simulink model "FOCSpdTrq"  (R2023a)
settings: Solver=ode1  StartTime=0.0  StopTime=0.2  FixedStep=ctrlConst.TsSwitch  MaxStep=1e-6  RelTol=1e-3  EnableMultiTasking=on
undefined symbols (not defined in the file or in its folder): ECM, f32_P_SpdNeglimit_rpm, f32_P_SpdPoslimit_rpm, f32_P_SpeedPiMaxRatio, f32_P_SpeedPiMinRatio, g_msgCore0to2_alphaLow, g_msgCore0to2_Asrctrlmode, g_msgCore0to2_AsrKpHi, g_msgCore0to2_AsrKpLo, g_msgCore0to2_AsrKpZero, g_msgCore0to2_AsrSwtHiRpm, g_msgCore0to2_AsrSwtLoRpm, g_msgCore0to2_AsrTiHi, g_msgCore0to2_AsrTiLo, g_msgCore0to2_AsrTiZero, g_msgCore0to2_betaLow, g_msgCore0to2_CalibEn2, g_msgCore0to2_coeff, g_msgCore0to2_cos_Amp, g_msgCore0to2_cos_frq, g_msgCore0to2_cos_phase, g_msgCore0to2_frqfix_K, g_msgCore0to2_H_coef, g_msgCore0to2_HFcoef, g_msgCore0to2_K1, g_msgCore0to2_K1switch, g_msgCore0to2_K2, g_msgCore0to2_K3, g_msgCore0to2_K3switch, g_msgCore0to2_Kvp, g_msgCore0to2_L_coef, g_msgCore0to2_LFcoef, g_msgCore0to2_LPF_coef, g_msgCore0to2_maxCur2, g_msgCore0to2_maxTrq2, g_msgCore0to2_R_Kr, g_msgCore0to2_R_outputGain, g_msgCore0to2_R_Outputlimit, g_msgCore0to2_R_Wc, g_msgCore0to2_Rswitch, g_msgCore0to2_sin_Amp, g_msgCore0to2_sin_frq, g_msgCore0to2_sin_phase, g_msgCore0to2_Trqfix, g_msgCoreoto2_R_woGain
libraries: simulink x2
settings Model: Creator=M00039784  LastModifiedBy=HP
settings SolverCC: AlgebraicLoopSolver=TrustRegion  InsertRTBMode=Never (minimum delay)
settings DataIOCC: LimitDataPoints=on  SaveFormat=Array  SaveOutput=off  SaveTime=off
settings OptimizationCC: DefaultParameterBehavior=Inlined  UseDivisionForNetSlopeComputation=on  UseFloatMulNetSlope=on  DefaultUnderspecifiedDataType=single  InlineInvariantSignals=on  ReuseModelBlockBuffer=off  PassReuseOutputArgsAs=Individual arguments  ExpressionDepthLimit=2147483647  ZeroExternalMemoryAtStartup=off  ZeroInternalMemoryAtStartup=off  NoFixptDivByZeroProtection=on  EfficientFloat2IntCast=on  LifeSpan=1  EfficientTunableParamExpr=on
settings DebuggingCC: ReadBeforeWriteMsg=DisableAll  WriteAfterWriteMsg=DisableAll  WriteAfterReadMsg=DisableAll  AlgebraicLoopMsg=none  MultiTaskDSMMsg=none  SingleTaskRateTransMsg=error  IntegerOverflowMsg=none  ParameterPrecisionLossMsg=none  BusObjectLabelMismatch=none  AssertControl=DisableAll  AllowSymbolicDim=off  StateNameClashWarn=warning  SFUnexpectedBacktrackingDiag=warning  SFNoUnconditionalDefaultTransitionDiag=warning  SFExecutionAtInitializationDiag=none  IntegerSaturationMsg=none  UnitsInconsistencyMsg=none  ArithmeticOperatorsInVariantConditions=warning
settings HardwareCC: ProdBitPerPointer=32  ProdBitPerSizeT=32  ProdBitPerPtrDiffT=32  ProdLargestAtomicFloat=None  ProdWordSize=32  ProdHWDeviceType=Infineon->TriCore
settings ModelReferenceCC: UpdateModelReferenceTargets=IfOutOfDate  EnableRefExpFcnMdlSchedulingChecks=on  ModelReferenceNumInstancesAllowed=Single  PropagateSignalLabelsOutOfModel=off
settings SFSimCC: SFSimEcho=off  SimUseLocalCustomCode=off  SimGenImportedTypeDefs=on  MATLABDynamicMemAlloc=off  CustomCodeUndefinedFunction=UseInterfaceOnly
settings RTWCC: Description=Embedded Coder  SystemTargetFile=ert.tlc  GenCodeOnly=on  GenerateMakefile=off  TemplateMakefile=ec_target.tmf  RTWVerbose=off  RTWUseLocalCustomCode=off  CodeExecutionProfiling=on  CodeProfilingSaveOptions=AllData  CodeProfilingInstrumentation=detailed
settings CodeAppCC: ForceParamTrailComments=on  IgnoreCustomStorageClasses=off  IgnoreTestpoints=on  MaxIdLength=64  SimulinkDataObjDesc=on  MATLABFcnDesc=on  CustomSymbolStrGlobalVar=GRS$N$M  CustomSymbolStrType=pmsmfocS_$N$M  CustomSymbolStrFcn=$N$M$F  CustomSymbolStrFcnArg=$I$N$M  CustomSymbolStrMacro=$N$M  InsertBlockDesc=on  StateflowObjectComments=on  MATLABSourceComments=on  InternalIdentifier=Classic
settings ERTTargetCC: TargetLangStandard=C99 (ISO)  UtilityFuncGeneration=Shared location  MultiwordLength=2048  CombineSignalStateStructs=on  SupportAbsoluteTime=off  SupportNonFinite=off  SupportComplex=off  SupportNonInlinedSFcns=on  RemoveResetFunc=off  ParenthesesLevel=Maximum  GenerateASAP2=on  InlinedParameterPlacement=NonHierarchical  ERTCustomFileTemplate=example_file_process.tlc  EnableDataOwnership=on  ConvertIfToSwitch=off  SuppressUnreachableDefaultCases=off  MemSecPackage=Simulink  MemSecDataConstants=MemConst  MemSecDataParameters=MemConstVolatile
settings ConfigComp: CovMetricSettings=dcmtrzow  CovHTMLOptions=-aTS=1 -bRG=1 -bTC=1 -hTR=0 -nFC=0 -scm=1 -bcm=1 -xEv=0  CovSaveCumulativeToWorkspaceVar=on  CovSaveSingleToWorkspaceVar=on  CovExternalEMLEnable=off  CovSFcnEnable=off
settings SimscapeCC: SimscapeNormalizeSystem=off

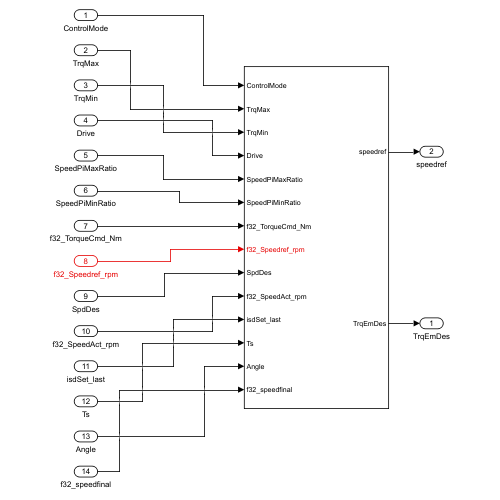
[thumbnail: Simulink's stored preview of the top-level diagram]
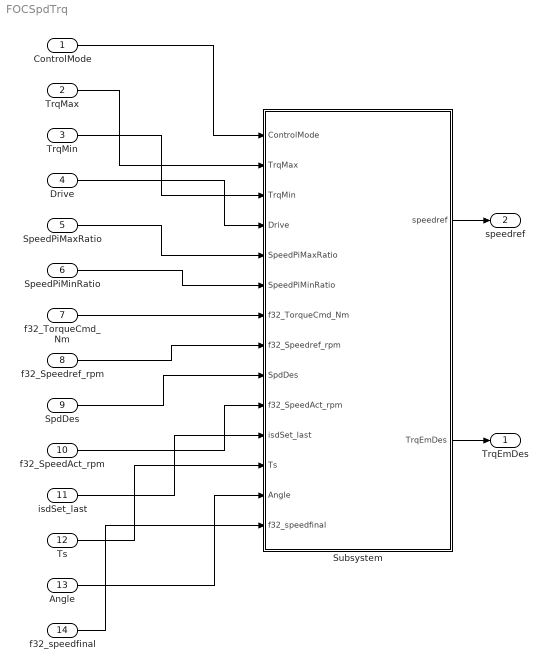
== system FOCSpdTrq ==
  ControlMode : Inport  OutDataTypeStr=Enum: ECM  PortDimensions=1  SampleTime=0.0001
  TrqMax : Inport  Port=2
  TrqMin : Inport  Port=3
  Drive : Inport  Port=4
  SpeedPiMaxRatio : Inport  Port=5
  SpeedPiMinRatio : Inport  Port=6
  f32_TorqueCmd_Nm : Inport  Port=7  OutDataTypeStr=single  PortDimensions=1
  f32_Speedref_rpm : Inport  Port=8  OutDataTypeStr=single  PortDimensions=1  SampleTime=0.0001
  SpdDes : Inport  Port=9
  f32_SpeedAct_rpm : Inport  Port=10  OutDataTypeStr=single  PortDimensions=1  SampleTime=0.0001
  isdSet_last : Inport  Port=11
  Ts : Inport  Port=12
  Angle : Inport  Port=13  OutDataTypeStr=int16  PortDimensions=1  SampleTime=0.0001
  f32_speedfinal : Inport  Port=14
  Subsystem : Subsystem
  TrqEmDes : Outport
  speedref : Outport  Port=2
  wires:
  SpeedPiMaxRatio/1 -> Subsystem/5(SpeedPiMaxRatio)
  SpdDes/1 -> Subsystem/9(SpdDes)
  ControlMode/1 -> Subsystem/1(ControlMode)
  SpeedPiMinRatio/1 -> Subsystem/6(SpeedPiMinRatio)
  TrqMax/1 -> Subsystem/2(TrqMax)
  f32_TorqueCmd_Nm/1 -> Subsystem/7(f32_TorqueCmd_Nm)
  TrqMin/1 -> Subsystem/3(TrqMin)
  f32_Speedref_rpm/1 -> Subsystem/8(f32_Speedref_rpm)
  Drive/1 -> Subsystem/4(Drive)
  f32_SpeedAct_rpm/1 -> Subsystem/10(f32_SpeedAct_rpm)
  isdSet_last/1 -> Subsystem/11(isdSet_last)
  Ts/1 -> Subsystem/12(Ts)
  Angle/1 -> Subsystem/13(Angle)
  f32_speedfinal/1 -> Subsystem/14(f32_speedfinal)
  Subsystem/1(speedref) -> speedref/1
  Subsystem/2(TrqEmDes) -> TrqEmDes/1

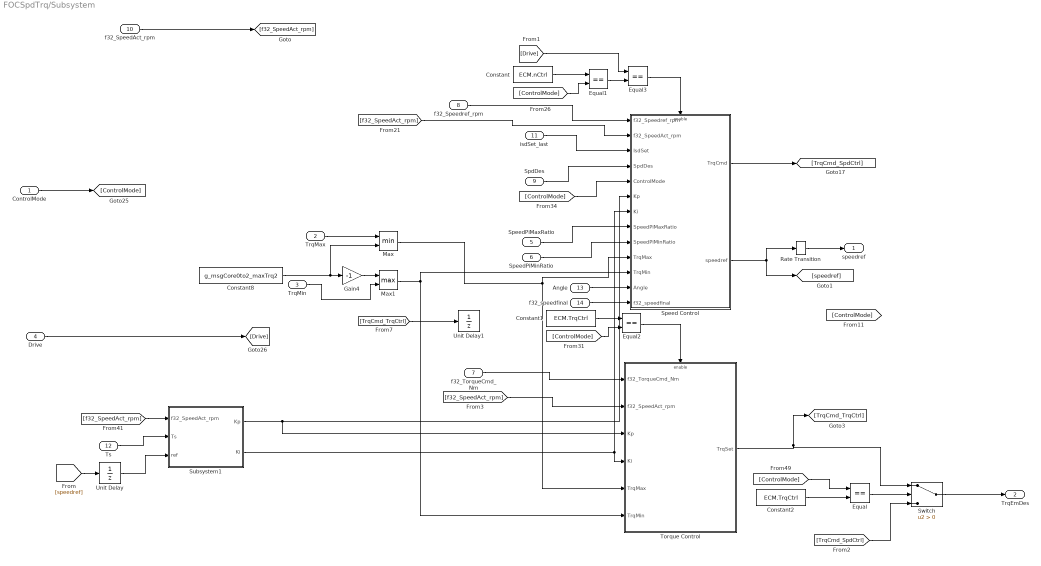
== system FOCSpdTrq/Subsystem ==
  ControlMode : Inport  OutDataTypeStr=Enum: ECM  PortDimensions=1  SampleTime=0.0001
  TrqMax : Inport  Port=2
  TrqMin : Inport  Port=3
  Drive : Inport  Port=4
  SpeedPiMaxRatio : Inport  Port=5
  SpeedPiMinRatio : Inport  Port=6
  f32_TorqueCmd_Nm : Inport  Port=7  OutDataTypeStr=single  PortDimensions=1
  f32_Speedref_rpm : Inport  Port=8  OutDataTypeStr=single  PortDimensions=1  SampleTime=0.0001
  SpdDes : Inport  Port=9
  f32_SpeedAct_rpm : Inport  Port=10  OutDataTypeStr=single  PortDimensions=1  SampleTime=0.0001
  isdSet_last : Inport  Port=11
  Ts : Inport  Port=12
  Angle : Inport  Port=13  OutDataTypeStr=int16  PortDimensions=1  SampleTime=0.0001
  f32_speedfinal : Inport  Port=14
  Constant : Constant  Value=ECM.nCtrl
  Constant1 : Constant  Value=ECM.TrqCtrl
  Constant2 : Constant  Value=ECM.TrqCtrl
  Constant8 : Constant  Value=g_msgCore0to2_maxTrq2  OutDataTypeStr=single  SampleTime=-1
  Equal{,1..3} (4 alike) : RelationalOperator  Operator===  OutDataTypeStr=boolean  RndMeth=Simplest  InputSameDT=off
  Gain4 : Gain  Gain=-1
  Max : MinMax  Inputs=2
  Max1 : MinMax  Function=max  Inputs=2
  Rate Transition : RateTransition
  Speed Control : Subsystem
  Subsystem1 : Subsystem
  Switch : Switch  Criteria=u2 > Threshold  SaturateOnIntegerOverflow=off  InputSameDT=off
  Torque Control : Subsystem
  Unit Delay : UnitDelay  SampleTime=-1  HasFrameUpgradeWarning=on
  Unit Delay1 : UnitDelay  SampleTime=-1  HasFrameUpgradeWarning=on
  speedref : Outport
  TrqEmDes : Outport  Port=2
  wires:
  isdSet_last/1 -> Speed Control/3(IsdSet)
  f32_Speedref_rpm/1 -> Speed Control/1(f32_Speedref_rpm)
  [ControlMode] -> Speed Control/5(ControlMode)
  Subsystem1/1(Kp) -> Speed Control/6(Kp), Torque Control/3(Kp)
  Equal1/1 -> Equal3/2
  Speed Control/1("TrqCmd ") -> [TrqCmd_SpdCtrl]
  Constant2/1 -> Equal/2
  SpeedPiMinRatio/1 -> Speed Control/9(SpeedPiMinRatio)
  [ControlMode] -> Equal/1
  Torque Control/1(TrqSet) -> Switch/1, [TrqCmd_TrqCtrl]
  Max/1 -> Speed Control/10(TrqMax), Torque Control/5(TrqMax)
  [Drive] -> Equal3/1
  Max1/1 -> Torque Control/6(TrqMin), Speed Control/11(TrqMin)
  [f32_SpeedAct_rpm] -> Speed Control/2(f32_SpeedAct_rpm)
  [f32_SpeedAct_rpm] -> Torque Control/2(f32_SpeedAct_rpm)
  SpeedPiMaxRatio/1 -> Speed Control/8(SpeedPiMaxRatio)
  Equal/1 -> Switch/2
  [ControlMode] -> Equal2/2
  Switch/1 -> TrqEmDes/1
  [ControlMode] -> Equal1/2
  TrqMin/1 -> Max1/2
  Subsystem1/2(Ki) -> Speed Control/7(Ki), Torque Control/4(Ki)
  ControlMode/1 -> [ControlMode]
  [TrqCmd_SpdCtrl] -> Switch/3
  Constant1/1 -> Equal2/1
  Drive/1 -> [Drive]
  [f32_SpeedAct_rpm] -> Subsystem1/1(f32_SpeedAct_rpm)
  Ts/1 -> Subsystem1/2(Ts)
  Constant/1 -> Equal1/1
  SpdDes/1 -> Speed Control/4(SpdDes)
  Equal2/1 -> Torque Control/Enable
  Gain4/1 -> Max1/1
  Constant8/1 -> Max/2, Gain4/1
  TrqMax/1 -> Max/1
  f32_SpeedAct_rpm/1 -> [f32_SpeedAct_rpm]
  Equal3/1 -> Speed Control/Enable
  Speed Control/2(speedref) -> Rate Transition/1, [speedref]
  f32_TorqueCmd_Nm/1 -> Torque Control/1(f32_TorqueCmd_Nm)
  [TrqCmd_TrqCtrl] -> Unit Delay1/1
  Angle/1 -> Speed Control/12(Angle)
  [speedref] -> Unit Delay/1
  Unit Delay/1 -> Subsystem1/3(ref)
  f32_speedfinal/1 -> Speed Control/13(f32_speedfinal)
  Rate Transition/1 -> speedref/1

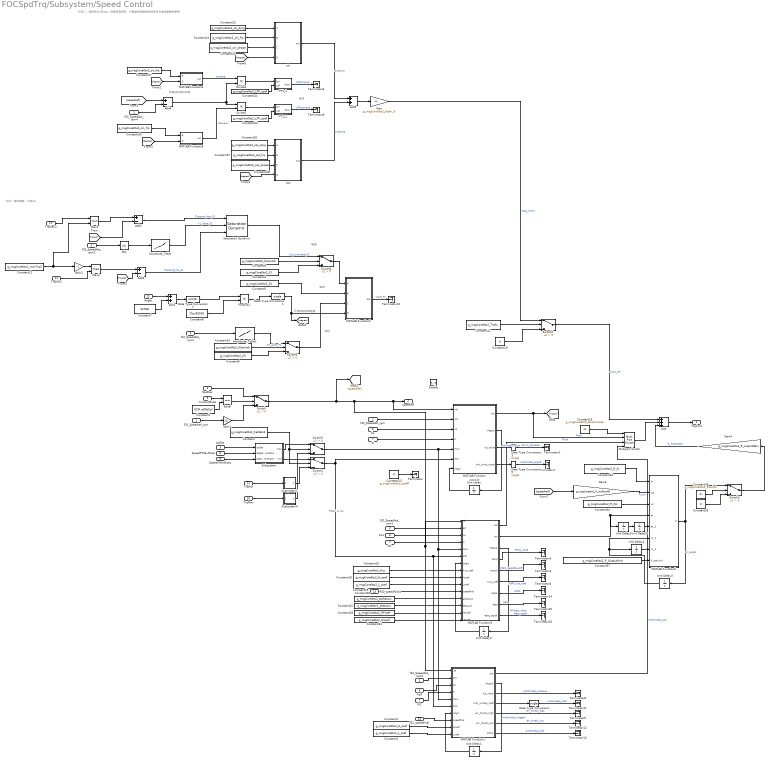
== system FOCSpdTrq/Subsystem/Speed Control ==
  note: PDFF & Up
  note: 幅值
  note: 方法二，同时有sin和cos，但是没有闭环，只把坐标变换后的信号作为调试参数的参考
  note: 方法一波动抑制，只有sin
  note: 去除系数
  note: 频率·
  note: 相位
  note: 外部接收机械角度
  note: 转速波动坐标变换
  note: 滤波
  f32_Speedref_rpm : Inport
  f32_SpeedAct_rpm : Inport  Port=2
  IsdSet : Inport  Port=3
  SpdDes : Inport  Port=4
  ControlMode : Inport  Port=5
  Kp : Inport  Port=6
  Ki : Inport  Port=7
  SpeedPiMaxRatio : Inport  Port=8
  SpeedPiMinRatio : Inport  Port=9
  TrqMax : Inport  Port=10
  TrqMin : Inport  Port=11
  Angle : Inport  Port=12  OutDataTypeStr=int16  PortDimensions=1  SampleTime=0.0001
  f32_speedfinal : Inport  Port=13
  Enable : EnablePort  StatesWhenEnabling=reset
  Abs : Abs  SaturateOnIntegerOverflow=off
  Add : Sum  Inputs=+++
  Add1 : Sum  OutDataTypeStr=int16
  Add2 : Sum  Inputs=+-
  Add3 : Sum  Inputs=+-
  Add4 : Sum  Inputs=+-
  Add5 : Sum
  Amplitude_Table : Lookup_n-D  NumberOfTableDimensions=1  DataSpecification=Lookup table object  LookupTableObject=cripple_T_P1  BreakpointsForDimension1=|  BeginIndexSearchUsingPreviousIndexResult=on  Table=|  ExtrapMethod=Clip  UseLastTableValue=on  InternalRulePriority=Speed  OutDataTypeStr=Inherit: Inherit from 'Table data'
      BreakpointsForDimension1=|
      | [-530.4101839
      | -495.049505
      | -459.688826
      | -424.3281471
      | -388.9674682
      | -353.6067893
      | -318.2461103
      | -282.8854314
      | -247.5247525
      | -212.1640736
      | -176.8033946
      | -141.4427157
      | -106.0820368
      | -70.72135785
      | -35.36067893
      | 0
      | 35.36067893
      | 70.72135785
      | 106.0820368
      | 141.4427157
      | 176.8033946
      | 212.1640736
      | 247.5247525
      | 282.8854314
      | 318.2461103
      | 353.6067893
      | 388.9674682
      | 424.3281471
      | 459.688826
      | 495.049505
      | 530.4101839
      | ]
      Table=|
      | [0.983333333
      | 0.983333333
      | 0.985185185
      | 0.987037037
      | 0.990740741
      | 0.992592593
      | 0.994444444
      | 0.996296296
      | 0.996296296
      | 0.998148148
      | 0.998148148
      | 0.998148148
      | 0.994444444
      | 0.992592593
      | 0.990740741
      | 0.990740741
      | 0.990740741
      | 0.992592593
      | 0.996296296
      | 1
      | 1
      | 1
      | 1
      | 0.998148148
      | 0.996296296
      | 0.994444444
      | 0.992592593
      | 0.990740741
      | 0.988888889
      | 0.987037037
      | 0.987037037]
  Amplitude_Table1 : Lookup_n-D  NumberOfTableDimensions=1  DataSpecification=Lookup table object  LookupTableObject=cphase_T_P1  BreakpointsForDimension1=|  BeginIndexSearchUsingPreviousIndexResult=on  Table=|  ExtrapMethod=Clip  UseLastTableValue=on  InternalRulePriority=Speed  OutDataTypeStr=Inherit: Inherit from 'Table data'
      BreakpointsForDimension1=|
      | [-530.4101839
      | -495.049505
      | -459.688826
      | -424.3281471
      | -388.9674682
      | -353.6067893
      | -318.2461103
      | -282.8854314
      | -247.5247525
      | -212.1640736
      | -176.8033946
      | -141.4427157
      | -106.0820368
      | -70.72135785
      | -35.36067893
      | 0
      | 35.36067893
      | 70.72135785
      | 106.0820368
      | 141.4427157
      | 176.8033946
      | 212.1640736
      | 247.5247525
      | 282.8854314
      | 318.2461103
      | 353.6067893
      | 388.9674682
      | 424.3281471
      | 459.688826
      | 495.049505
      | 530.4101839
      | ]
      Table=|
      | [0.983333333
      | 0.983333333
      | 0.985185185
      | 0.987037037
      | 0.990740741
      | 0.992592593
      | 0.994444444
      | 0.996296296
      | 0.996296296
      | 0.998148148
      | 0.998148148
      | 0.998148148
      | 0.994444444
      | 0.992592593
      | 0.990740741
      | 0.990740741
      | 0.990740741
      | 0.992592593
      | 0.996296296
      | 1
      | 1
      | 1
      | 1
      | 0.998148148
      | 0.996296296
      | 0.994444444
      | 0.992592593
      | 0.990740741
      | 0.988888889
      | 0.987037037
      | 0.987037037]
  Constant : Constant  Value=g_msgCore0to2_CalibEn2
  Constant1 : Constant  Value=g_msgCore0to2_H_coef
  Constant10 : Constant  Value=0  OutDataTypeStr=single
  Constant11 : Constant  Value=g_msgCore0to2_Trqfix  OutDataTypeStr=single
  Constant12 : Constant  Value=g_msgCore0to2_maxTrq2  OutDataTypeStr=single  SampleTime=-1
  Constant13 : Constant  Value=g_msgCore0to2_coeff  OutDataTypeStr=single
  Constant14 : Constant  Value=g_msgCore0to2_K3switch
  Constant15 : Constant  Value=g_msgCore0to2_Kvp
  Constant16 : Constant  Value=g_msgCore0to2_Asrctrlmode
  Constant17 : Constant  Value=g_msgCore0to2_sin_frq
  Constant18 : Constant  Value=g_msgCore0to2_H_coef
  Constant19 : Constant  Value=g_msgCore0to2_L_coef
  Constant2 : Constant  Value=ECM.alOfsCal
  Constant20 : Constant  Value=g_msgCore0to2_alphaLow
  Constant21 : Constant  Value=g_msgCore0to2_LPF_coef  OutDataTypeStr=single
  Constant22 : Constant  Value=g_msgCore0to2_LPF_coef  OutDataTypeStr=single
  Constant23 : Constant  Value=g_msgCore0to2_sin_Amp
  Constant24 : Constant  Value=g_msgCore0to2_sin_frq
  Constant25 : Constant  Value=g_msgCore0to2_sin_phase
  Constant26 : Constant  Value=g_msgCore0to2_cos_Amp
  Constant27 : Constant  Value=g_msgCore0to2_cos_frq
  Constant28 : Constant  Value=g_msgCore0to2_cos_phase
  Constant29 : Constant  Value=g_msgCore0to2_HFcoef
  Constant3 : Constant  Value=g_msgCore0to2_L_coef
  Constant30 : Constant  Value=g_msgCore0to2_sin_frq
  Constant31 : Constant  Value=g_msgCore0to2_LFcoef
  Constant32 : Constant  Value=g_msgCore0to2_betaLow
  Constant33 : Constant  Value=g_msgCore0to2_R_Kr
  Constant34 : Constant  Value=g_msgCore0to2_R_Wc
  Constant35 : Constant  Value=0
  Constant36 : Constant  Value=g_msgCore0to2_Rswitch
  Constant37 : Constant  Value=g_msgCore0to2_R_Outputlimit
  Constant4 : Constant  Value=g_msgCore0to2_K1
  Constant5 : Constant  Value=g_msgCore0to2_K2
  Constant6 : Constant  Value=g_msgCore0to2_K3
  Constant7 : Constant  Value=32768  OutDataTypeStr=int16
  Constant8 : Constant  Value=2*pi/65535  OutDataTypeStr=single
  Constant9 : Constant  Value=g_msgCore0to2_K1switch
  Data Type Conversion{,1,3,5} (4 alike) : DataTypeConversion  OutDataTypeStr=single  SaturateOnIntegerOverflow=off  RndMeth=Floor
  Data Type Conversion2 : DataTypeConversion  OutDataTypeStr=uint16  SaturateOnIntegerOverflow=off  RndMeth=Floor
  Divide1 : Product  Inputs=**  OutDataTypeStr=single
  Divide2 : Product  Inputs=**  OutDataTypeStr=single
  Equal : RelationalOperator  Operator===  OutDataTypeStr=boolean  RndMeth=Simplest  InputSameDT=off
  Gain : Gain  Gain=g_msgCore0to2_frqfix_K
  Gain1 : Gain  Gain=12
  Gain2 : Gain  Gain=-1
  Gain3 : Gain  Gain=g_msgCoreoto2_R_woGain/60
  Gain4 : Gain  Gain=g_msgCore0to2_R_outputGain  OutDataTypeStr=single
  Ki1 : InportShadow  Port=7
  Ki2 : InportShadow  Port=7
  Kp1 : InportShadow  Port=6
  Kp3 : InportShadow  Port=6
  MATLAB Function : MATLAB Function  TreatAsAtomicUnit=on
  MATLAB Function1 : MATLAB Function  TreatAsAtomicUnit=on
  MATLAB Function2 : MATLAB Function  TreatAsAtomicUnit=on
  MATLAB Function3 : MATLAB Function  TreatAsAtomicUnit=on
  MATLAB Function4 : MATLAB Function  TreatAsAtomicUnit=on
  MATLAB Function5 : MATLAB Function  TreatAsAtomicUnit=on
  MATLAB Function6 : MATLAB Function  TreatAsAtomicUnit=on
  Max2 : MinMax  Inputs=2
  Max3 : MinMax  Function=max  Inputs=2
  Multiport Switch : MultiPortSwitch  SaturateOnIntegerOverflow=off  InputSameDT=off
  PT1_1 : Subsystem
  PT1_2 : Subsystem
  Product1 : Product  OutDataTypeStr=single
  Saturation Dynamic : simulink/Discontinuities/Saturation Dynamic  OutMin=[]  OutMax=[]  OutDataTypeStr=Inherit: Same as second input  OutDataType=fixdt(1, 16)  OutScaling=2^-10  DoSatur=off
  Subsystem : Subsystem
  Subsystem1 : Subsystem
  Subsystem4 : Subsystem
  Switch{,1..6} (7 alike) : Switch  Criteria=u2 > Threshold  SaturateOnIntegerOverflow=off  InputSameDT=off
  Terminator{,1..16} (17 alike) : Terminator
  TrqMax2 : InportShadow  Port=10
  TrqMin2 : InportShadow  Port=11
  Unit Delay{,1..6} (7 alike) : UnitDelay  SampleTime=-1  HasFrameUpgradeWarning=on
  cos : MATLAB Function  TreatAsAtomicUnit=on
  f32_SpeedAct_rpm{1..5} (5 alike) : InportShadow  Port=2
  f32_speedfinal1 : InportShadow  Port=13
  "sin " : MATLAB Function  TreatAsAtomicUnit=on
  "TrqCmd " : Outport  OutputWhenDisabled=reset  InitialOutput=0
  speedref : Outport  Port=2  OutputWhenDisabled=reset  InitialOutput=0
  wires:
  IsdSet/1 -> Subsystem/1(IsdSet)
  Switch2/1 -> MATLAB Function/6(MIN), MATLAB Function1/6(MIN), MATLAB Function3/6(MIN)
  Switch1/1 -> MATLAB Function/5(MAX), MATLAB Function1/5(MAX), MATLAB Function3/5(MAX)
  f32_SpeedAct_rpm/1 -> MATLAB Function/2(act)
  Switch/1 -> [speedref], MATLAB Function1/1(ref), MATLAB Function3/1(ref), MATLAB Function/1(ref), speedref/1
  MATLAB Function/2(intgout) -> Unit Delay/1  "Asrintgin_value"
  ControlMode/1 -> Equal/1
  Equal/1 -> Switch/2
  SpdDes/1 -> Switch/1
  f32_Speedref_rpm/1 -> Gain1/1
  Constant2/1 -> Equal/2
  Gain1/1 -> Switch/3
  Kp/1 -> MATLAB Function/3(kp)
  Ki/1 -> MATLAB Function/4(ki)
  SpeedPiMaxRatio/1 -> Subsystem/2(SpeedPiMaxRatio)
  SpeedPiMinRatio/1 -> Subsystem/3(SpeedPiMinRatio)
  Subsystem/1(max) -> Switch1/1
  Subsystem/2(min) -> Switch2/1
  Constant/1 -> Switch1/2, Switch2/2
  TrqMin/1 -> Subsystem1/1(" ")
  TrqMax/1 -> Subsystem4/1(" ")
  Subsystem4/1(Outport) -> Switch1/3
  Subsystem1/1(Outport) -> Switch2/3
  Unit Delay/1 -> MATLAB Function/7(intgin)
  Switch6/1 -> MATLAB Function2/3(C)
  Max3/1 -> Add3/1
  Constant12/1 -> Gain2/1, Max2/2
  Saturation Dynamic/1 -> Switch4/1  "K1_Limitvalue_P1"
  f32_SpeedAct_rpm3/1 -> Abs/1
  [Trqspd] -> Add2/2
  Amplitude_Table/1 -> Saturation Dynamic/2  "K1_value_P1"
  Add3/1 -> Saturation Dynamic/3  "Trqcomp_Min_P1"
  [Trqspd] -> Add3/2
  Switch5/1 -> Add/1  "comp_P1"
  Max2/1 -> Add2/1
  Constant9/1 -> Switch4/2
  Constant14/1 -> Switch6/2
  Constant8/1 -> Product1/2
  Constant7/1 -> Add1/2
  Constant6/1 -> Switch6/3
  TrqMin2/1 -> Max3/2
  Constant4/1 -> Switch4/3
  Gain2/1 -> Max3/1
  Constant10/1 -> Switch5/3
  Constant5/1 -> MATLAB Function2/2(B)
  Add2/1 -> Saturation Dynamic/1  "Trqcomp_Max_P1"
  Angle/1 -> Add1/1
  Abs/1 -> Amplitude_Table/1
  Constant11/1 -> Switch5/2
  Data Type Conversion1/1 -> [degree], MATLAB Function2/4(D)
  f32_SpeedAct_rpm2/1 -> Amplitude_Table1/1
  Product1/1 -> Data Type Conversion1/1
  Amplitude_Table1/1 -> Switch6/1  "K3_value_P1"
  Switch4/1 -> MATLAB Function2/1(A)
  Add1/1 -> Data Type Conversion2/1
  Data Type Conversion2/1 -> Product1/1
  Add/1 -> "TrqCmd "/1
  TrqMax2/1 -> Max2/1
  MATLAB Function/1(out) -> Multiport Switch/2, [Trqspd]  "PIout"
  MATLAB Function/3(Kp_value) -> Data Type Conversion3/1
  Constant16/1 -> Multiport Switch/1
  MATLAB Function3/1(out) -> Multiport Switch/3  "FFout"
  MATLAB Function3/3(intgout) -> Unit Delay2/1  "FFintgin_value"
  Unit Delay2/1 -> MATLAB Function3/7(intgin)
  f32_SpeedAct_rpm1/1 -> MATLAB Function3/2(act)
  Ki1/1 -> MATLAB Function3/4(ki)
  Kp1/1 -> MATLAB Function3/3(kp)
  Data Type Conversion3/1 -> Terminator1/1  "AsrKp_Calvalue"
  MATLAB Function3/4(temp) -> Terminator3/1  "FFKp_value"
  [speedref] -> Add4/1
  f32_SpeedAct_rpm4/1 -> Add4/2
  [degree] -> MATLAB Function4/2(D)
  [degree] -> MATLAB Function5/2(D)
  MATLAB Function4/1(out) -> Divide1/1  "sinwave"
  Add4/1 -> Divide2/1, Divide1/2
  MATLAB Function5/1(out) -> Divide2/2  "coswave"
  Divide1/1 -> PT1_1/1(bin)
  Constant21/1 -> PT1_1/2(cof)
  Divide2/1 -> PT1_2/1(bin)
  Constant22/1 -> PT1_2/2(cof)
  "sin "/1(out) -> Add5/1  "sinfixtrq"
  cos/1(out) -> Add5/2  "cosfixtrq"
  Add5/1 -> Gain/1
  [degree] -> cos/4(D)
  [degree] -> "sin "/4(D)
  Constant23/1 -> "sin "/1(A)
  Constant24/1 -> "sin "/2(B)
  Constant25/1 -> "sin "/3(C)
  Constant26/1 -> cos/1(A)
  Constant27/1 -> cos/2(B)
  Constant28/1 -> cos/3(C)
  Constant17/1 -> MATLAB Function4/1(B)
  Constant30/1 -> MATLAB Function5/1(B)
  Gain/1 -> Switch5/1  "total_fixtrq"
  Constant13/1 -> Terminator/1
  PT1_1/1(bout) -> Terminator6/1  "LPFsinwave"
  PT1_2/1(bout) -> Terminator9/1  "LPFcoswave"
  MATLAB Function2/1(out) -> Terminator10/1  "wave_P1"
  Kp3/1 -> MATLAB Function1/3(kp)
  Ki2/1 -> MATLAB Function1/4(ki)
  f32_SpeedAct_rpm5/1 -> MATLAB Function1/2(act)
  Unit Delay1/1 -> MATLAB Function1/7(intgin)
  MATLAB Function1/2(intgout) -> Unit Delay1/1  "AntiWindup_integral"
  MATLAB Function1/3(Kp_value) -> Terminator8/1  "AntiWindup_Kpvalue"
  MATLAB Function1/4(Anti_windup_coef) -> Data Type Conversion/1
  Data Type Conversion/1 -> Terminator11/1  "AntiWindup_coef"
  Multiport Switch/1 -> Add/2
  MATLAB Function1/1(out) -> Multiport Switch/4  "AntiWindup_out"
  MATLAB Function/4(Anti_wind_signal) -> Data Type Conversion5/1
  Data Type Conversion5/1 -> Terminator7/1  "AntiWindup_Signal"
  f32_speedfinal/1 -> MATLAB Function1/8(speedfinal)
  Constant1/1 -> MATLAB Function1/9(Hcoef)
  Constant3/1 -> MATLAB Function1/10(Lcoef)
  MATLAB Function1/5(err_thresh_high) -> Terminator5/1  "err_thresh_high"
  MATLAB Function1/6(err_thresh_low) -> Terminator12/1  "err_thresh_low"
  MATLAB Function1/7(alpha) -> Terminator13/1  "AntiWindup_Alfa"
  MATLAB Function3/5(temp1) -> Terminator2/1  "PDFF_SpdrefMuxKff"
  MATLAB Function3/6(Kvp_coef) -> Terminator4/1  "PDFF_Kvp_coef"
  Constant15/1 -> MATLAB Function3/8("Kvp_coef ")
  Constant18/1 -> MATLAB Function3/9(Hcoef)
  Constant19/1 -> MATLAB Function3/10(Lcoef)
  f32_speedfinal1/1 -> MATLAB Function3/11(speedfinal)
  Constant20/1 -> MATLAB Function3/12(alphaLow)
  MATLAB Function3/7(alpha) -> Terminator14/1  "alpha"
  Constant32/1 -> MATLAB Function3/13(betaLow)
  Constant29/1 -> MATLAB Function3/14(HFcoef)
  Constant31/1 -> MATLAB Function3/15(LFcoef)
  MATLAB Function3/8(beta) -> Terminator15/1  "beta"
  MATLAB Function3/9(beta_signal) -> Terminator16/1  "beta_signal"
  MATLAB Function6/1(yk) -> Unit Delay3/1, Switch3/1  "R_output"
  Unit Delay4/1 -> MATLAB Function6/7(yk_2)
  Unit Delay3/1 -> Unit Delay4/1, MATLAB Function6/6(yk_1)
  MATLAB Function3/2(err) -> Unit Delay6/1, MATLAB Function6/4(ek)
  Unit Delay5/1 -> MATLAB Function6/5(ek_2)
  Unit Delay6/1 -> Unit Delay5/1
  [speedref] -> Gain3/1
  Gain3/1 -> MATLAB Function6/2(w0)  "R_wo"
  Constant33/1 -> MATLAB Function6/1(Kr)
  Constant34/1 -> MATLAB Function6/3(wc)
  Switch3/1 -> Gain4/1
  Constant35/1 -> Switch3/3
  Constant36/1 -> Switch3/2
  Gain4/1 -> Add/3  "R_finaloutput"
  Constant37/1 -> MATLAB Function6/8(R_optLimt)

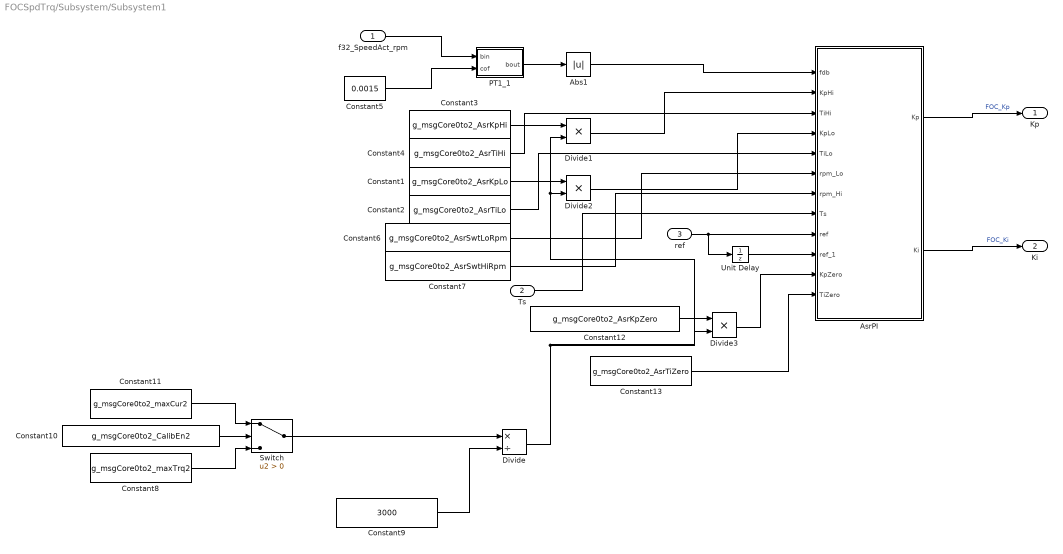
== system FOCSpdTrq/Subsystem/Subsystem1 ==
  f32_SpeedAct_rpm : Inport
  Ts : Inport  Port=2
  ref : Inport  Port=3
  Abs1 : Abs  SaturateOnIntegerOverflow=off
  AsrPI : MATLAB Function
  Constant1 : Constant  Value=g_msgCore0to2_AsrKpLo
  Constant10 : Constant  Value=g_msgCore0to2_CalibEn2
  Constant11 : Constant  Value=g_msgCore0to2_maxCur2  OutDataTypeStr=single  SampleTime=-1
  Constant12 : Constant  Value=g_msgCore0to2_AsrKpZero
  Constant13 : Constant  Value=g_msgCore0to2_AsrTiZero
  Constant2 : Constant  Value=g_msgCore0to2_AsrTiLo
  Constant3 : Constant  Value=g_msgCore0to2_AsrKpHi
  Constant4 : Constant  Value=g_msgCore0to2_AsrTiHi
  Constant5 : Constant  Value=0.0015  OutDataTypeStr=single
  Constant6 : Constant  Value=g_msgCore0to2_AsrSwtLoRpm
  Constant7 : Constant  Value=g_msgCore0to2_AsrSwtHiRpm
  Constant8 : Constant  Value=g_msgCore0to2_maxTrq2  OutDataTypeStr=single  SampleTime=-1
  Constant9 : Constant  Value=3000  OutDataTypeStr=single  SampleTime=-1
  Divide : Product  Inputs=*/  OutDataTypeStr=single
  Divide1 : Product  Inputs=**  OutDataTypeStr=single
  Divide2 : Product  Inputs=**  OutDataTypeStr=single
  Divide3 : Product  Inputs=**  OutDataTypeStr=single
  PT1_1 : Subsystem
  Switch : Switch  Criteria=u2 > Threshold  SaturateOnIntegerOverflow=off  InputSameDT=off
  Unit Delay : UnitDelay  SampleTime=-1  HasFrameUpgradeWarning=on
  Kp : Outport
  Ki : Outport  Port=2
  wires:
  f32_SpeedAct_rpm/1 -> PT1_1/1(bin)
  Constant5/1 -> PT1_1/2(cof)
  PT1_1/1(bout) -> Abs1/1
  Abs1/1 -> AsrPI/1(fdb)
  Constant4/1 -> AsrPI/3(TiHi)
  Constant2/1 -> AsrPI/5(TiLo)
  Constant6/1 -> AsrPI/6(rpm_Lo)
  Constant7/1 -> AsrPI/7(rpm_Hi)
  Ts/1 -> AsrPI/8(Ts)
  AsrPI/1(Kp) -> Kp/1  "FOC_Kp"
  AsrPI/2(Ki) -> Ki/1  "FOC_Ki"
  Constant9/1 -> Divide/2
  Constant3/1 -> Divide1/1
  Divide/1 -> Divide3/2, Divide2/2, Divide1/2
  Divide1/1 -> AsrPI/2(KpHi)
  Constant1/1 -> Divide2/1
  Divide2/1 -> AsrPI/4(KpLo)
  Constant10/1 -> Switch/2
  Constant11/1 -> Switch/1
  Switch/1 -> Divide/1
  Constant8/1 -> Switch/3
  ref/1 -> Unit Delay/1, AsrPI/9(ref)
  Unit Delay/1 -> AsrPI/10(ref_1)
  Constant13/1 -> AsrPI/12(TiZero)
  Constant12/1 -> Divide3/1
  Divide3/1 -> AsrPI/11(KpZero)

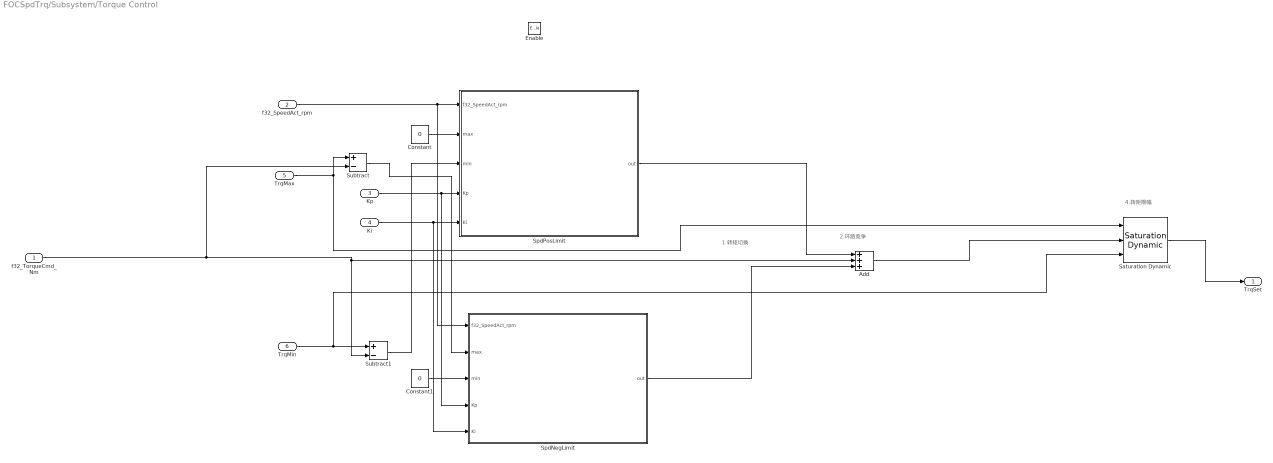
== system FOCSpdTrq/Subsystem/Torque Control ==
  note: 4.转矩限幅
  note: 1.转矩切换
  note: 2.环路竞争
  f32_TorqueCmd_Nm : Inport
  f32_SpeedAct_rpm : Inport  Port=2
  Kp : Inport  Port=3
  Ki : Inport  Port=4
  TrqMax : Inport  Port=5
  TrqMin : Inport  Port=6
  Enable : EnablePort  StatesWhenEnabling=reset
  Add : Sum  Inputs=+++
  Constant : Constant  Value=0  OutDataTypeStr=single
  Constant1 : Constant  Value=0  OutDataTypeStr=single
  Saturation Dynamic : simulink/Discontinuities/Saturation Dynamic  OutMin=[]  OutMax=[]  OutDataTypeStr=Inherit: Same as second input  OutDataType=fixdt(1, 16)  OutScaling=2^-10  DoSatur=off
  SpdNegLimit : Subsystem
  SpdPosLimit : Subsystem
  Subtract : Sum  Inputs=+-
  Subtract1 : Sum  Inputs=+-
  TrqSet : Outport  OutputWhenDisabled=reset  InitialOutput=0  VectorParamsAs1DForOutWhenUnconnected=off
  wires:
  Saturation Dynamic/1 -> TrqSet/1
  TrqMax/1 -> Subtract/1, Saturation Dynamic/1
  TrqMin/1 -> Saturation Dynamic/3, Subtract1/1
  Subtract/1 -> SpdNegLimit/2(max)
  Subtract1/1 -> SpdPosLimit/3(min)
  SpdPosLimit/1(out) -> Add/1
  SpdNegLimit/1(out) -> Add/3
  Kp/1 -> SpdNegLimit/4(Kp), SpdPosLimit/4(Kp)
  Ki/1 -> SpdNegLimit/5(Ki), SpdPosLimit/5(Ki)
  f32_SpeedAct_rpm/1 -> SpdPosLimit/1(f32_SpeedAct_rpm), SpdNegLimit/1(f32_SpeedAct_rpm)
  Constant/1 -> SpdPosLimit/2(max)
  Constant1/1 -> SpdNegLimit/3(min)
  f32_TorqueCmd_Nm/1 -> Subtract1/2, Add/2, Subtract/2
  Add/1 -> Saturation Dynamic/2

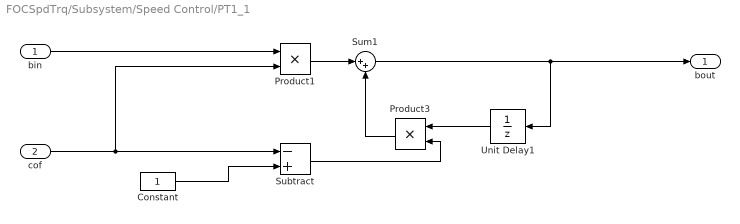
== system FOCSpdTrq/Subsystem/Speed Control/PT1_1 ==
  bin : Inport
  cof : Inport  Port=2
  Constant : Constant  OutDataTypeStr=single
  Product1 : Product  RndMeth=Zero  OutDataTypeStr=Inherit: Same as first input
  Product3 : Product  RndMeth=Zero  OutDataTypeStr=Inherit: Same as first input
  Subtract : Sum  Inputs=-+  OutDataTypeStr=Inherit: Same as first input
  Sum1 : Sum  Inputs=|++  OutDataTypeStr=Inherit: Same as first input
  Unit Delay1 : UnitDelay  SampleTime=-1  HasFrameUpgradeWarning=on
  bout : Outport  VectorParamsAs1DForOutWhenUnconnected=off
  wires:
  Product3/1 -> Sum1/2
  Unit Delay1/1 -> Product3/1
  Product1/1 -> Sum1/1
  bin/1 -> Product1/1
  Constant/1 -> Subtract/2
  cof/1 -> Subtract/1, Product1/2
  Sum1/1 -> bout/1, Unit Delay1/1
  Subtract/1 -> Product3/2

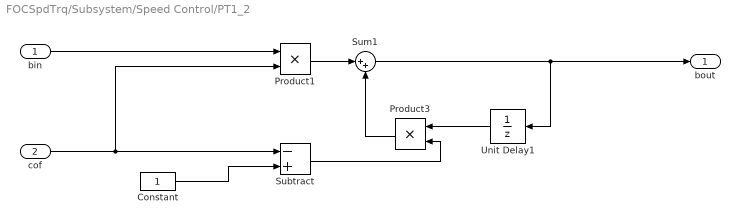
== system FOCSpdTrq/Subsystem/Speed Control/PT1_2 ==
  bin : Inport
  cof : Inport  Port=2
  Constant : Constant  OutDataTypeStr=single
  Product1 : Product  RndMeth=Zero  OutDataTypeStr=Inherit: Same as first input
  Product3 : Product  RndMeth=Zero  OutDataTypeStr=Inherit: Same as first input
  Subtract : Sum  Inputs=-+  OutDataTypeStr=Inherit: Same as first input
  Sum1 : Sum  Inputs=|++  OutDataTypeStr=Inherit: Same as first input
  Unit Delay1 : UnitDelay  SampleTime=-1  HasFrameUpgradeWarning=on
  bout : Outport  VectorParamsAs1DForOutWhenUnconnected=off
  wires:
  Product3/1 -> Sum1/2
  Unit Delay1/1 -> Product3/1
  Product1/1 -> Sum1/1
  bin/1 -> Product1/1
  Constant/1 -> Subtract/2
  cof/1 -> Subtract/1, Product1/2
  Sum1/1 -> bout/1, Unit Delay1/1
  Subtract/1 -> Product3/2

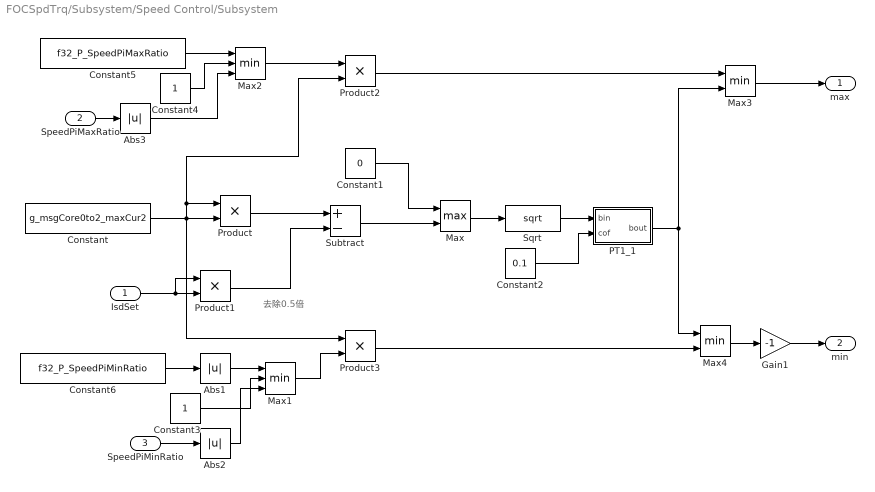
== system FOCSpdTrq/Subsystem/Speed Control/Subsystem ==
  note: 去除0.5倍
  IsdSet : Inport
  SpeedPiMaxRatio : Inport  Port=2
  SpeedPiMinRatio : Inport  Port=3
  Abs1 : Abs  SaturateOnIntegerOverflow=off
  Abs2 : Abs  SaturateOnIntegerOverflow=off
  Abs3 : Abs  SaturateOnIntegerOverflow=off
  Constant : Constant  Value=g_msgCore0to2_maxCur2
  Constant1 : Constant  Value=0  OutDataTypeStr=single
  Constant2 : Constant  Value=0.1  OutDataTypeStr=single
  Constant3 : Constant  OutDataTypeStr=single
  Constant4 : Constant  OutDataTypeStr=single
  Constant5 : Constant  Value=f32_P_SpeedPiMaxRatio
  Constant6 : Constant  Value=f32_P_SpeedPiMinRatio
  Gain1 : Gain  Gain=-1
  Max : MinMax  Function=max  Inputs=2
  Max1 : MinMax  Inputs=3
  Max2 : MinMax  Inputs=3
  Max3 : MinMax  Inputs=2
  Max4 : MinMax  Inputs=2
  PT1_1 : Subsystem
  Product{,1..3} (4 alike) : Product
  Sqrt : Sqrt
  Subtract : Sum  Inputs=+-
  max : Outport  VectorParamsAs1DForOutWhenUnconnected=off
  min : Outport  Port=2  VectorParamsAs1DForOutWhenUnconnected=off
  wires:
  Gain1/1 -> min/1
  Sqrt/1 -> PT1_1/1(bin)
  Max/1 -> Sqrt/1
  Constant1/1 -> Max/1
  Subtract/1 -> Max/2
  Product1/1 -> Subtract/2
  IsdSet/1 -> Product1/2, Product1/1
  Product/1 -> Subtract/1
  Constant/1 -> Product3/1, Product2/2, Product/1, Product/2
  PT1_1/1(bout) -> Max3/2, Max4/1
  Constant2/1 -> PT1_1/2(cof)
  Constant6/1 -> Abs1/1
  Abs1/1 -> Max1/1
  Constant3/1 -> Max1/2
  Constant5/1 -> Max2/1
  Constant4/1 -> Max2/2
  Max2/1 -> Product2/1
  Max1/1 -> Product3/2
  Product2/1 -> Max3/1
  Max3/1 -> max/1
  Product3/1 -> Max4/2
  Max4/1 -> Gain1/1
  SpeedPiMinRatio/1 -> Abs2/1
  SpeedPiMaxRatio/1 -> Abs3/1
  Abs2/1 -> Max1/3
  Abs3/1 -> Max2/3

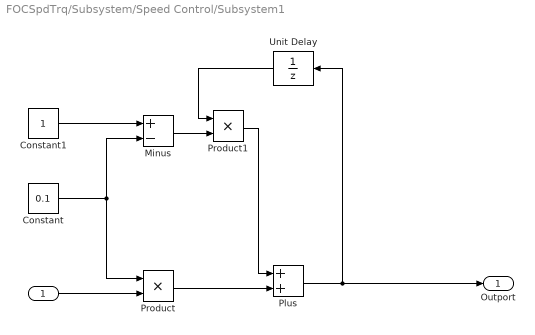
== system FOCSpdTrq/Subsystem/Speed Control/Subsystem1 ==
  " " : Inport
  Constant : Constant  Value=0.1  OutDataTypeStr=single
  Constant1 : Constant  OutDataTypeStr=single
  Minus : Sum  Inputs=+-
  Plus : Sum
  Product : Product
  Product1 : Product
  Unit Delay : UnitDelay  SampleTime=-1  HasFrameUpgradeWarning=on
  Outport : Outport
  wires:
  Product/1 -> Plus/2
  Unit Delay/1 -> Product1/1
  Constant1/1 -> Minus/1
  Product1/1 -> Plus/1
  Minus/1 -> Product1/2
  Constant/1 -> Product/1, Minus/2
  " "/1 -> Product/2
  Plus/1 -> Unit Delay/1, Outport/1

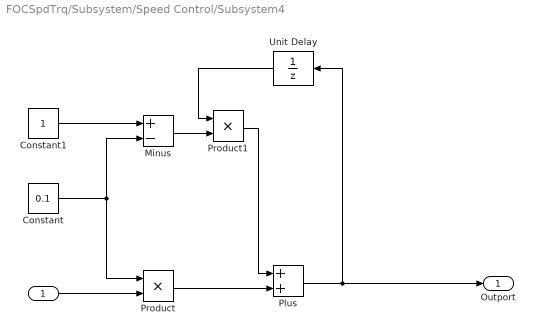
== system FOCSpdTrq/Subsystem/Speed Control/Subsystem4 ==
  " " : Inport
  Constant : Constant  Value=0.1  OutDataTypeStr=single
  Constant1 : Constant  OutDataTypeStr=single
  Minus : Sum  Inputs=+-
  Plus : Sum
  Product : Product
  Product1 : Product
  Unit Delay : UnitDelay  SampleTime=-1  HasFrameUpgradeWarning=on
  Outport : Outport
  wires:
  Plus/1 -> Outport/1, Unit Delay/1
  " "/1 -> Product/2
  Constant/1 -> Minus/2, Product/1
  Minus/1 -> Product1/2
  Product1/1 -> Plus/1
  Constant1/1 -> Minus/1
  Unit Delay/1 -> Product1/1
  Product/1 -> Plus/2

== system FOCSpdTrq/Subsystem/Subsystem1/PT1_1 ==
  bin : Inport
  cof : Inport  Port=2
  Constant : Constant  OutDataTypeStr=single
  Product1 : Product  RndMeth=Zero  OutDataTypeStr=Inherit: Same as first input
  Product3 : Product  RndMeth=Zero  OutDataTypeStr=Inherit: Same as first input
  Subtract : Sum  Inputs=-+  OutDataTypeStr=Inherit: Same as first input
  Sum1 : Sum  Inputs=|++  OutDataTypeStr=Inherit: Same as first input
  Unit Delay1 : UnitDelay  SampleTime=-1  HasFrameUpgradeWarning=on
  bout : Outport  VectorParamsAs1DForOutWhenUnconnected=off
  wires:
  Product3/1 -> Sum1/2
  Unit Delay1/1 -> Product3/1
  Product1/1 -> Sum1/1
  bin/1 -> Product1/1
  Constant/1 -> Subtract/2
  cof/1 -> Subtract/1, Product1/2
  Sum1/1 -> bout/1, Unit Delay1/1
  Subtract/1 -> Product3/2

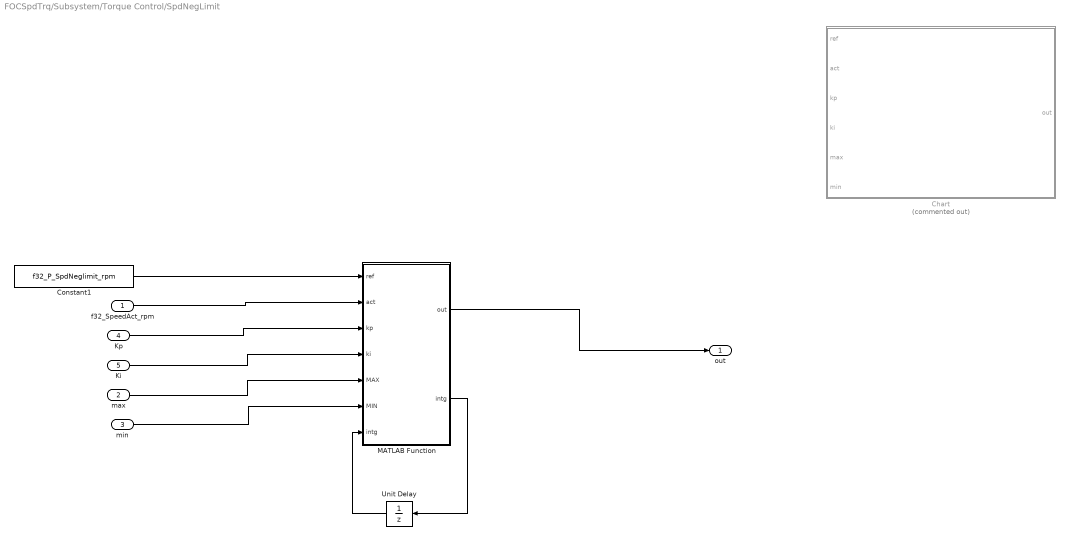
== system FOCSpdTrq/Subsystem/Torque Control/SpdNegLimit ==
  f32_SpeedAct_rpm : Inport
  max : Inport  Port=2
  min : Inport  Port=3
  Kp : Inport  Port=4
  Ki : Inport  Port=5
  Chart : Stateflow chart  Commented=on  TreatAsAtomicUnit=on
  Constant1 : Constant  Value=f32_P_SpdNeglimit_rpm
  MATLAB Function : MATLAB Function  TreatAsAtomicUnit=on
  Unit Delay : UnitDelay  SampleTime=-1  HasFrameUpgradeWarning=on
  out : Outport  VectorParamsAs1DForOutWhenUnconnected=off
  wires:
  MATLAB Function/1(out) -> out/1
  Kp/1 -> MATLAB Function/3(kp)
  max/1 -> MATLAB Function/5(MAX)
  Ki/1 -> MATLAB Function/4(ki)
  f32_SpeedAct_rpm/1 -> MATLAB Function/2(act)
  min/1 -> MATLAB Function/6(MIN)
  Constant1/1 -> MATLAB Function/1(ref)
  Unit Delay/1 -> MATLAB Function/7("intg ")
  MATLAB Function/2(intg) -> Unit Delay/1

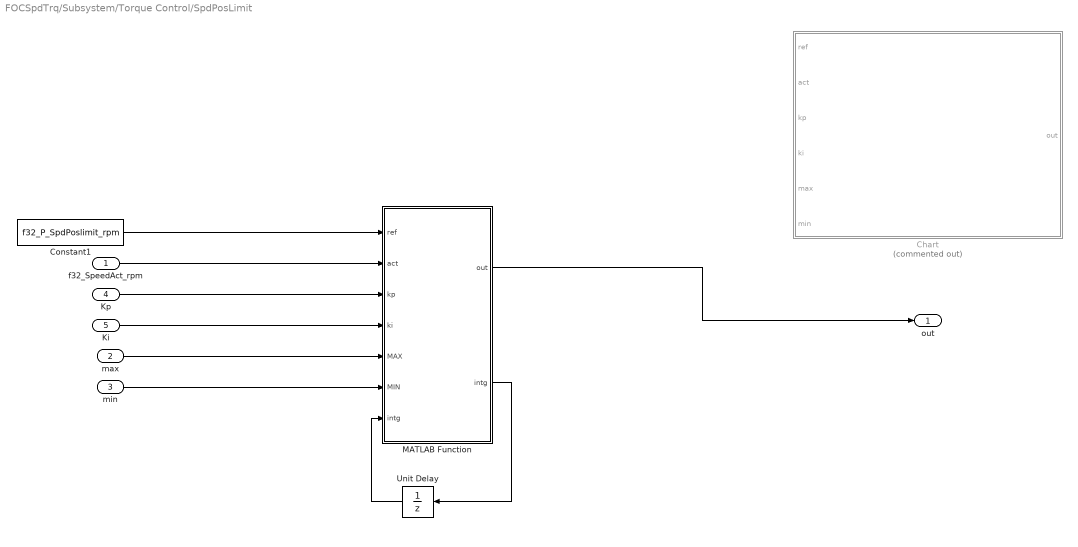
== system FOCSpdTrq/Subsystem/Torque Control/SpdPosLimit ==
  f32_SpeedAct_rpm : Inport
  max : Inport  Port=2
  min : Inport  Port=3
  Kp : Inport  Port=4
  Ki : Inport  Port=5
  Chart : Stateflow chart  Commented=on  TreatAsAtomicUnit=on
  Constant1 : Constant  Value=f32_P_SpdPoslimit_rpm
  MATLAB Function : MATLAB Function  TreatAsAtomicUnit=on
  Unit Delay : UnitDelay  SampleTime=-1  HasFrameUpgradeWarning=on
  out : Outport  VectorParamsAs1DForOutWhenUnconnected=off
  wires:
  max/1 -> MATLAB Function/5(MAX)
  Constant1/1 -> MATLAB Function/1(ref)
  f32_SpeedAct_rpm/1 -> MATLAB Function/2(act)
  Kp/1 -> MATLAB Function/3(kp)
  Ki/1 -> MATLAB Function/4(ki)
  MATLAB Function/1(out) -> out/1
  Unit Delay/1 -> MATLAB Function/7("intg ")
  MATLAB Function/2(intg) -> Unit Delay/1
  min/1 -> MATLAB Function/6(MIN)

== system FOCSpdTrq/Subsystem/Speed Control/Subsystem/PT1_1 ==
  bin : Inport
  cof : Inport  Port=2
  Constant : Constant  OutDataTypeStr=single
  Product1 : Product  RndMeth=Zero  OutDataTypeStr=Inherit: Same as first input
  Product3 : Product  RndMeth=Zero  OutDataTypeStr=Inherit: Same as first input
  Subtract : Sum  Inputs=-+  OutDataTypeStr=Inherit: Same as first input
  Sum1 : Sum  Inputs=|++  OutDataTypeStr=Inherit: Same as first input
  Unit Delay1 : UnitDelay  SampleTime=-1  HasFrameUpgradeWarning=on
  bout : Outport  VectorParamsAs1DForOutWhenUnconnected=off
  wires:
  Product3/1 -> Sum1/2
  Unit Delay1/1 -> Product3/1
  Product1/1 -> Sum1/1
  bin/1 -> Product1/1
  Constant/1 -> Subtract/2
  cof/1 -> Subtract/1, Product1/2
  Sum1/1 -> bout/1, Unit Delay1/1
  Subtract/1 -> Product3/2

== matlab function FOCSpdTrq/Subsystem/Speed Control/MATLAB Function4 ==
  data: B input; out output; D input
function out  = fcn(B,D)


out = sin(B*D);

== matlab function FOCSpdTrq/Subsystem/Speed Control/MATLAB Function5 ==
  data: B input; out output; D input
function out  = fcn(B,D)
out = cos(B*D);

== matlab function FOCSpdTrq/Subsystem/Speed Control/sin  ==
  data: A input; out output; B input; C input; D input
function out  = fcn(A,B,C,D)


out = A*sin(B*D+C);

== matlab function FOCSpdTrq/Subsystem/Speed Control/MATLAB Function6 ==
  data: Kr input; yk output; w0 input; wc input; ek input; ek_2 input; yk_1 input; yk_2 input; R_optLimt input
function yk = fcn(Kr,w0, wc,ek,ek_2,yk_1,yk_2,R_optLimt)

Ts = 1/16000;

b=(4+4*wc*Ts+w0^2*Ts^2);

b0=(4*Kr*wc*Ts)/b;
b2=(-4*Kr*wc*Ts)/b;
a1=(2*w0^2*Ts^2-8)/b;
a2=(4-4*wc*Ts+w0^2*Ts^2)/b;

yk = b0*ek+b2*ek_2-a1*yk_1-a2*yk_2;




out_limt = R_optLimt;
if yk>out_limt
    yk=out_limt;
elseif yk<-out_limt
    yk=-out_limt;
end
end

== matlab function FOCSpdTrq/Subsystem/Speed Control/cos ==
  data: A input; out output; B input; C input; D input
function out  = fcn(A,B,C,D)


out = A*cos(B*D+C);

== matlab function FOCSpdTrq/Subsystem/Speed Control/MATLAB Function ==
  data: ref input; out output; act input; kp input; ki input; MAX input; MIN input; intgin input single; intgout output; Kp_value output; Anti_wind_signal output
function [out,intgout,Kp_value,Anti_wind_signal] = fcn(ref,act,kp,ki,MAX,MIN,intgin)
err = (ref - act);    %去除系数
Kp_value = err*kp;

temp = err*kp;
out = temp + intgin;


if(out>MAX)
    out = MAX;
    Anti_wind_signal =single(0);
    if(err<0)
        intgin = intgin + ki*err;
        Anti_wind_signal =single(1);
    end
elseif(out < MIN)
        out = MIN;
        Anti_wind_signal =single(0);

        if(err>0)
            intgin = intgin + ki*err;
            Anti_wind_signal =single(1);
        end
else
    intgin = intgin + ki*err;
    Anti_wind_signal =single(0);
end
max(intgin,MIN);
min(intgin,MAX);
intgout = intgin;

== stateflow chart FOCSpdTrq/Subsystem/Torque Control/SpdNegLimit/Chart ==
  state PID
    en:
    err=0;
    integ=0;
    du:
    err=ref-act;
    out=kp*err+integ;
    if out>max
    out=max;
    if(err<0)
    integ=integ+ki*err;
    end
    elseif out<min
    out=min;
    if(err>0)
    integ=integ+ki*err;
    end
    else
    integ=integ+ki*err;
    end
    if integ>max
    integ=max;
    elseif integ <min
    integ=min;
    end
  (default) -> PID
  data: ref input single; act input single; kp input single; ki input single; out output single; integ local single; max input single; min input single; err local single

== matlab function FOCSpdTrq/Subsystem/Torque Control/SpdNegLimit/MATLAB Function ==
  data: ref input; out output; act input; kp input; ki input; MAX input; MIN input; intg input single; intg output
function [out,intg]  = fcn(ref,act,kp,ki,MAX,MIN,intg)
persistent temp;
err = ref - act;
temp = err*kp;
out = temp + intg;
if(out>MAX)
    out = MAX;
    if(err<0)
        intg = intg + ki*err;
    end
elseif(out < MIN)
        out = MIN;
        if(err>0)
            intg = intg + ki*err;
        end
else
    intg = intg + ki*err;
end
max(intg,MIN);
min(intg,MAX);

== stateflow chart FOCSpdTrq/Subsystem/Torque Control/SpdPosLimit/Chart ==
  state PID
    en:
    err=0;
    integ=0;
    du:
    err=ref-act;
    out=kp*err+integ;
    if out>max
    out=max;
    if(err<0)
    integ=integ+ki*err;
    end
    elseif out<min
    out=min;
    if(err>0)
    integ=integ+ki*err;
    end
    else
    integ=integ+ki*err;
    end
    if integ>max
    integ=max;
    elseif integ <min
    integ=min;
    end
  (default) -> PID
  data: ref input single; act input single; kp input single; ki input single; out output single; integ local single; max input single; min input single; err local single

== matlab function FOCSpdTrq/Subsystem/Torque Control/SpdPosLimit/MATLAB Function ==
  data: ref input; out output; act input; kp input; ki input; MAX input; MIN input; intg input single; intg output
function [out,intg] = fcn(ref,act,kp,ki,MAX,MIN,intg)
err = ref - act;
temp = err*kp;
out = temp + intg;
if(out>MAX)
    out = MAX;
    if(err<0)
        intg = intg + ki*err;
    end
elseif(out < MIN)
        out = MIN;
        if(err>0)
            intg = intg + ki*err;
        end
else
    intg = intg + ki*err;
end
max(intg,MIN);
min(intg,MAX);

== matlab function FOCSpdTrq/Subsystem/Subsystem1/AsrPI ==
  data: Kp output single; Ki output single; fdb input; KpHi input; TiHi input; KpLo input; TiLo input; rpm_Lo input; rpm_Hi input; Ts input; ref input; ref_1 input; KpZero input; TiZero input
function [Kp,Ki]   = fcn(fdb,KpHi,TiHi,KpLo,TiLo,rpm_Lo,rpm_Hi,Ts,ref,ref_1,KpZero,TiZero)
%
if TiHi == single(0)
    asrKiHi = single(0);
else
    asrKiHi = KpHi*Ts/TiHi;
end

if TiLo == single(0)
    asrKiLo = single(0);
else
    asrKiLo = KpLo*Ts/TiLo;
end

if rpm_Hi >= rpm_Lo
    asr_rpm_Hi = rpm_Hi;
    asr_rpm_Lo = rpm_Lo;
else
    asr_rpm_Hi = rpm_Lo;
    asr_rpm_Lo = rpm_Hi;
end

if fdb >= asr_rpm_Hi
    Kp = KpHi;
    Ki = asrKiHi;
elseif fdb <= asr_rpm_Lo
    Kp = KpLo;
    Ki = asrKiLo;
else
    Kp = (KpHi - KpLo)*(fdb - asr_rpm_Lo)/(asr_rpm_Hi - asr_rpm_Lo) + KpLo;
    Ki = (asrKiHi - asrKiLo)*(fdb - asr_rpm_Lo)/(asr_rpm_Hi - asr_rpm_Lo) + asrKiLo;
end

if (ref == 0) && (ref_1 ==0)
    Kp = KpZero;
    Ki = KpZero*Ts/TiZero;
end

== matlab function FOCSpdTrq/Subsystem/Speed Control/MATLAB Function1 ==
  data: ref input; out output; act input; kp input; ki input; MAX input; MIN input; intgin input single; intgout output; Kp_value output; Anti_windup_coef output; speedfinal input; Hcoef input; Lcoef input; err_thresh_high output; err_thresh_low output; alpha output
function [out,intgout,Kp_value,Anti_windup_coef,err_thresh_high,err_thresh_low,alpha] = fcn(ref,act,kp,ki,MAX,MIN,intgin,speedfinal,Hcoef,Lcoef)
err = (ref - act);    %去除系数
Kp_value = err*kp;

temp = Kp_value + intgin;

if(temp>MAX)
    out = MAX;
elseif(temp < MIN)
    out = MIN;   
else
    out = temp;
end

Anti_windup_coef = abs(temp -out);

err_thresh_high = speedfinal *Hcoef ;
err_thresh_low = speedfinal * Lcoef;


    err_abs = abs(err);
    if(err_abs > err_thresh_high)
    alpha = single(0.0);          % 大误差：完全关积分
    elseif(err_abs < err_thresh_low)
    alpha = single(1.0);          % 小误差：全开积分
    else
    % 线性平滑过渡，彻底消除开关抖动
    alpha = single((err_thresh_high - err_abs)/(err_thresh_high - err_thresh_low));
    end

  if(abs(speedfinal)<300)
   alpha = single(1);
  end

if(Anti_windup_coef > single(0))
    intgin =  out - Kp_value;
else
    %intgin = intgin + ki*err;
    intgin = intgin + alpha * ki * err;
end

% max(intgin,MIN);
% min(intgin,MAX);
intgout = intgin;

== matlab function FOCSpdTrq/Subsystem/Speed Control/MATLAB Function2 ==
  data: A input; out output; B input; C input; D input
function out  = fcn(A,B,C,D)


out = A*sin(B*D+C);

== matlab function FOCSpdTrq/Subsystem/Speed Control/MATLAB Function3 ==
  data: ref input; out output; err output; act input; kp input; ki input; MAX input; MIN input; intgin input single; intgout output; Kvp_coef input; temp output; temp1 output; Kvp_coef output; Hcoef input; Lcoef input; speedfinal input; alphaLow input; alpha output; betaLow input; HFcoef input; LFcoef input; beta output; beta_signal output
function [out,err,intgout,temp,temp1,Kvp_coef,alpha,beta,beta_signal] = fcn(ref,act,kp,ki,MAX,MIN,intgin,Kvp_coef,Hcoef,Lcoef,speedfinal,alphaLow,betaLow,HFcoef,LFcoef)
%%%%%%%%%%%% KVP取值约为0.001-0.005 
err = (ref - act);    %去除系数
temp = err*kp;


%%PDFF要折算

err_thresh_high = speedfinal *Hcoef ;
err_thresh_low = speedfinal * Lcoef;
err_abs = abs(err);
if(err_abs > err_thresh_high)
alpha = single(alphaLow);          % 大误差：不能完全关积分
elseif(err_abs < err_thresh_low)
alpha = single(1.0);          % 小误差：全开积分
else
% 线性平滑过渡，彻底消除开关抖动
alpha = single(((err_thresh_high - err_abs)*(single(1.0)-single(alphaLow)))/(err_thresh_high - err_thresh_low)) +  single(alphaLow) ;
end


PDFF_high =  single(7000)*HFcoef ;
PDFF_low = single(7000)* LFcoef;

if(abs(speedfinal) >PDFF_high) %%如果转速大于某个值
beta = single(betaLow);         %%要缩小PDFF系数
beta_signal =single(0);
elseif(abs(speedfinal) < PDFF_low)  %%如果小于某个值，保持不变  这样在低速下可以用较大的pdff系数
beta = single(1.0);  
beta_signal =single(1);
else
% 线性平滑过渡，彻底消除开关抖动
beta = single(((PDFF_high - abs(speedfinal))*(single(1.0)-single(betaLow)))/(PDFF_high - PDFF_low)) +  single(betaLow) ;
beta_signal =single(2);
end


%Kvp = kp *Kvp_coef*beta;
Kvp = kp *Kvp_coef*beta;
temp1=Kvp*act;
out = temp + intgin-temp1;
    

if(out>MAX)
    out = MAX;
    if(err<0)
        intgin = intgin + ki*err;
    end
elseif(out < MIN)
        out = MIN;
        if(err>0)
            intgin = intgin + ki*err;
        end
else
    intgin = intgin + alpha*ki*err;
   %intgin = intgin + ki*err;
end

%----------------------------------------------------------------------------%

max(intgin,MIN);
min(intgin,MAX);
intgout = intgin;
